simulink model "monopod_controller"  (R2022a)
settings: Solver=FixedStepDiscrete  StartTime=0.0  StopTime=10.0  FixedStep=1/f_c  RelTol=1e-3
values from neighbouring files (symbols this model uses):
  g = 9.81    [monopod_controller_parameter.sldd]
  I_1 = 0.1    [monopod_controller_parameter.sldd]
  I_2 = 0.1    [monopod_controller_parameter.sldd]
  I_body = 0.1    [monopod_controller_parameter.sldd]
  l_1 = 0.16    [monopod_controller_parameter.sldd]
  l_2 = 0.16    [monopod_controller_parameter.sldd]
  m_1 = 0.158    [monopod_controller_parameter.sldd]
  m_2 = 0.062    [monopod_controller_parameter.sldd]
  m_body = 0.1    [monopod_controller_parameter.sldd]
  trq_max = 2.7    [monopod_controller_parameter.sldd]
settings Model: DataDictionary=monopod_controller_parameter.sldd  EnableAccessToBaseWorkspace=off  Creator=chris  LastModifiedBy=chris

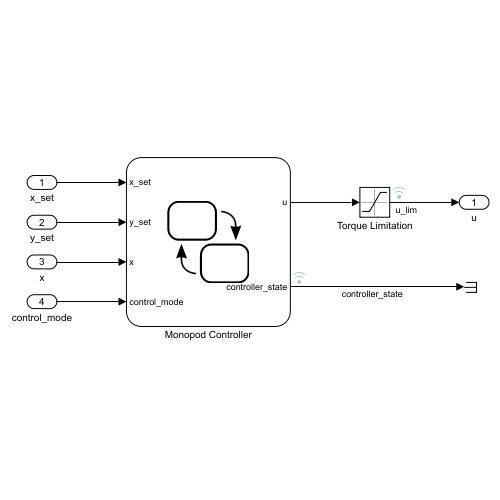
[thumbnail: Simulink's stored preview of the top-level diagram]
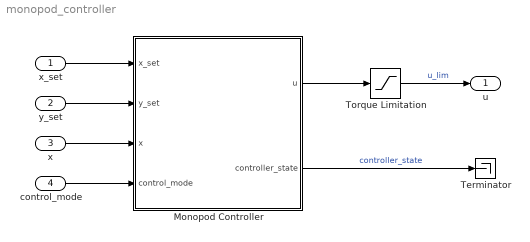
== system monopod_controller ==
  x_set : Inport
  y_set : Inport  Port=2
  x : Inport  Port=3
  control_mode : Inport  Port=4
  Monopod Controller : Stateflow chart  TreatAsAtomicUnit=on
  Terminator : Terminator
  Torque Limitation : Saturate  UpperLimit=trq_max  LowerLimit=-trq_max
  u : Outport
  wires:
  x_set/1 -> Monopod Controller/1(x_set)
  Monopod Controller/2(controller_state) -> Terminator/1  "controller_state"
  x/1 -> Monopod Controller/3(x)
  Monopod Controller/1(u) -> Torque Limitation/1
  control_mode/1 -> Monopod Controller/4(control_mode)
  y_set/1 -> Monopod Controller/2(y_set)
  Torque Limitation/1 -> u/1  "u_lim"

== stateflow chart monopod_controller/Monopod Controller ==
  state Thrust_Phase
    entry:
    controller_state = 3
    lambda = get_lambda(x,u);
    thrust_profile = hopping_height_controller(y_set, y_apex)
    i = 1;
    during:
    lambda = get_lambda(x,u);
    u = thrust2torque(thrust_profile(i));
    i = i+1;
  state Flight_Phase
    entry:
    controller_state = 0;
    y_foot = get_c(0,x);
    y_apex =  x(1);
    during:
    y_foot = get_c(0,x);
    y_apex = max(x(1), y_apex);
    u = impedance_controller(x_set, x, 2);
  state Stance_Phase
    entry:
    controller_state = 2;
    lambda = get_lambda(x,u);
    during:
    lambda = get_lambda(x,u);
    u = impedance_controller(x_set, x, 2);
  state Impact_Phase
    entry:
    controller_state = 1;
  Stance_Phase -> Thrust_Phase [order 2] : [ abs(x(4)) < 0.01 && control_mode==1 ]
  Thrust_Phase -> Flight_Phase [order 1] : [ lambda(2) == 0 && i == length(thrust_profile) ]
  Thrust_Phase -> Stance_Phase [order 2] : [ lambda(2) ~= 0 && i == length(thrust_profile) ]
  (default) -> Flight_Phase
  Stance_Phase -> Flight_Phase [order 1] : [ lambda(2) == 0 ]
  Impact_Phase -> Stance_Phase
  Flight_Phase -> Impact_Phase : [ y_foot <= 0]
  data: thrust function_input; u_new function_output; x_set input size=[2,1]; y_set input; y_foot local; u output size=[2,1] =[0;0]; x input size=[6,1]; controller_state output; y_apex local; control_mode input; thrust_profile local; i local; lambda local; I_1 parameter; I_2 parameter; I_body parameter; l_1 parameter; l_2 parameter; m_1 parameter; m_2 parameter; m_body parameter; g parameter
  data control_mode settings: description=|
      | 0 = impedance control
      | 1 = hopping height control
  function u_new = thrust2torque(thrust):
    | function u_new = thrust2torque(thrust)
    |     F_p = [0; thrust];
    |     J_pq = get_J_pq(x);
    |     u_new = transpose(J_pq) * F_p;
    | end
